simulink subsystem "DriveControl"  (R2023a)
settings: Solver=VariableStepAuto  StartTime=0.0  StopTime=10.0  RelTol=1e-3
settings Model: Creator=Franz  LastModifiedBy=Franz

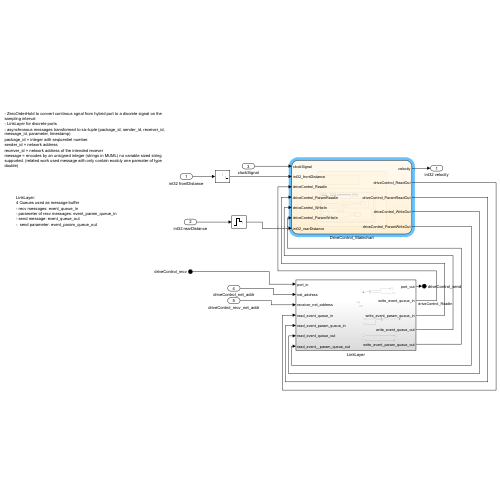
[thumbnail: Simulink's stored preview of the top-level diagram]
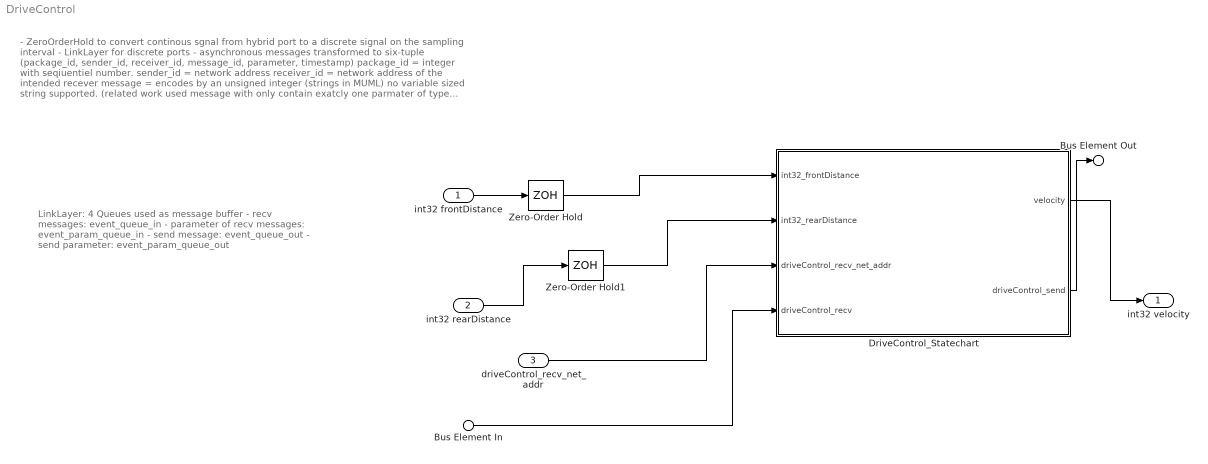
== system DriveControl ==
  note: LinkLayer:
      | 4 Queues used as message buffer
      | - recv messages: event_queue_in
      | - parameter of recv messages: event_param_queue_in
      | - send message: event_queue_out
      | -  send parameter: event_param_queue_out
  note: - ZeroOrderHold to convert continous sgnal from hybrid port to a discrete signal on the sampling interval
      | - LinkLayer for discrete ports
      | - asynchronous messages transformed to six-tuple (package_id, sender_id, receiver_id, message_id, parameter, timestamp)
      | package_id = integer with seqiuentiel number.
      | sender_id = network address
      | receiver_id = network address of the intended recever
      | message = encodes by an unsigned integer (strings in MUML) no variable sized string supported. (related work used message with only contain exatcly one parmater of type double)
  int32 frontDistance : Inport  OutDataTypeStr=int32
  int32 rearDistance : Inport  Port=2  OutDataTypeStr=int32
  driveControl_recv_net_addr : Inport  Port=3
  Bus Element In : Inport  Port=4  PortName=driveControl_recv
  DriveControl_Statechart : Stateflow chart  TreatAsAtomicUnit=on
  Zero-Order Hold : ZeroOrderHold  SampleTime=30
  Zero-Order Hold1 : ZeroOrderHold  SampleTime=30
  int32 velocity : Outport  OutDataTypeStr=int32
  Bus Element Out : Outport  Port=2  PortName=driveControl_send
  wires:
  DriveControl_Statechart/1(velocity) -> int32 velocity/1
  Zero-Order Hold/1 -> DriveControl_Statechart/1(int32_frontDistance)
  int32 frontDistance/1 -> Zero-Order Hold/1
  int32 rearDistance/1 -> Zero-Order Hold1/1
  Zero-Order Hold1/1 -> DriveControl_Statechart/2(int32_rearDistance)
  Bus Element In/1 -> DriveControl_Statechart/4(driveControl_recv)
  driveControl_recv_net_addr/1 -> DriveControl_Statechart/3(driveControl_recv_net_addr)
  DriveControl_Statechart/2(driveControl_send) -> Bus Element Out/1

== stateflow chart DriveControl/DriveControl_Statechart ==
  note: initial state in MUML: add default state
      | parallel: direct child-states can be active in parallel (dashed boderline)
      | exclusive: only one child can be active (solid borderline)
      | region to parallel states
  state chart
    state chartRegion [parallel]
      settings: executionOrder=1
      state DriveControlComponent
        state driveControlport [parallel]
          settings: executionOrder=2
          state AutonomusDriving
          state WaitForPermission
          state Overtaking
          AutonomusDriving -> WaitForPermission : requestPermission[int32_frontDistance<distanceLimit]{velocity = 50 }
          (default) -> AutonomusDriving
          WaitForPermission -> AutonomusDriving [order 2] : denyPermission
          Overtaking -> AutonomusDriving : overtakingSuccessful
          WaitForPermission -> Overtaking [order 1] : grantPermission{accelerate; send(startOvertaking); driveControl_send = 1}
        state driving [parallel]
          settings: executionOrder=1
          state PassSlowerVehicle
          note: Do action are not considered by the transformation
          state FollowMainLane
          state CompleteOvertaking
          (default) -> FollowMainLane
          PassSlowerVehicle -> CompleteOvertaking
          FollowMainLane -> PassSlowerVehicle : startOvertaking{changeLaneLeft;}
          CompleteOvertaking -> FollowMainLane : [int32_rearDistance > 2 * distanceLimit]{changeLaneRight; send(overtakingSuccessful)}
      (default) -> DriveControlComponent
  (default) -> chart
  data: distanceLimit constant int32 =10; int32_frontDistance input; int32_rearDistance input; velocity output; driveControl_recv_net_addr input; driveControl_recv input; driveControl_send output
  events: overtakingSuccessful local FUNCTION_CALL_EVENT; startOvertaking local FUNCTION_CALL_EVENT; executedOvertaking local FUNCTION_CALL_EVENT; denyPermission local FUNCTION_CALL_EVENT; grantPermission local RISING_EDGE_EVENT; requestPermission local FUNCTION_CALL_EVENT
  function changeLaneRight:
    | function changeLaneRight
  function slowVelocity:
    | function slowVelocity
  function changeLaneLeft:
    | function changeLaneLeft
  function accelerate:
    | function accelerate
